simulink model "k6jca_181230_SHERA_ARDUINO_Comparison"  (R2018b)
settings: Solver=ode45  StartTime=0.0  StopTime=9000  MaxStep=1  RelTol=1e-3  EnableMultiTasking=on
InitFcn:
  | D=30
settings Model: Creator=Dick  LastModifiedBy=Jeff
settings DataIOCC: LimitDataPoints=on  SaveFormat=Array  SaveOutput=off  SignalLogging=off  DSMLogging=off  SaveTime=off
settings OptimizationCC: LifeSpan=inf
settings DebuggingCC: SFUnexpectedBacktrackingDiag=warning  SFNoUnconditionalDefaultTransitionDiag=warning  SFExecutionAtInitializationDiag=none
settings HardwareCC: ProdBitPerPointer=32  ProdBitPerSizeT=32  ProdBitPerPtrDiffT=32  ProdLargestAtomicFloat=None  ProdIntDivRoundTo=Undefined  ProdEndianess=Unspecified  ProdWordSize=32  ProdHWDeviceType=32-bit Generic
settings ModelReferenceCC: PropagateSignalLabelsOutOfModel=off
settings SFSimCC: SimUseLocalCustomCode=off
settings RTWCC: RTWUseLocalCustomCode=off
settings CodeAppCC: StateflowObjectComments=on
settings GRTTargetCC: TargetLangStandard=C89/C90 (ANSI)  GeneratePreprocessorConditionals=Disable all
settings ConfigComp: CovMetricSettings=dw  CovHtmlReporting=on  CovSaveCumulativeToWorkspaceVar=on  CovSaveSingleToWorkspaceVar=on  CovExternalEMLEnable=off

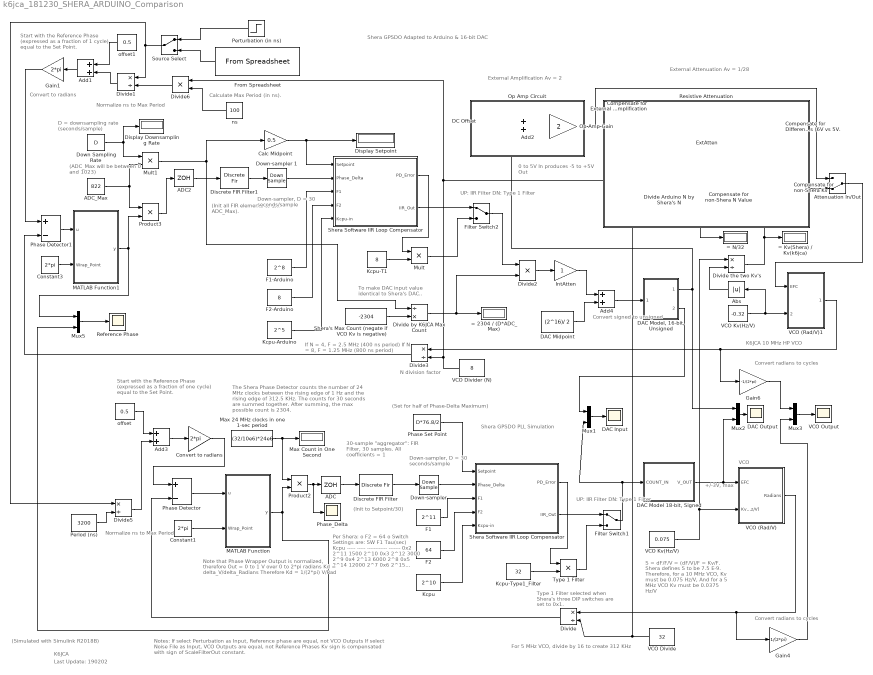
== system k6jca_181230_SHERA_ARDUINO_Comparison ==
  note: (Simulated with Simulink R2018B)
  note: Convert
      | signed
      | to unsigned
  note: To make DAC input value
      | identical to Shera's DAC..
  note: Notes:
      | If select Perturbation as Input, Reference phase are equal, not VCO Outputs
      | If select Noise File as Input, VCO Outputs are equal, not Reference Phases
      | Kv sign is compensated with sign of ScaleFilterOut constant.
  note: Normalize ns to
      | Max Period
  note: Calculate Max Period
      | (in ns).
  note: Down-sampler,
      | D = 30
      | seconds/sample
  note: Last Update: 190202
  note: (Set for half of Phase-Delta Maximum)
  note: 30-sample "aggregator":
      | FIR Filter,
      | 30 samples.
      | All coefficients = 1
  note: Start with the Reference Phase
      | (expressed as a fraction of one cycle)
      | equal to the Set Point.
  note: UP:  IIR Filter
      | DN:  Type 1 Filter
  note: Type 1 Filter selected
      | when Shera's three
      | DIP switches are set to 0x1.
  note: S = dF/F/V = (dF/V)/F = Kv/F.
      | Shera defines S to be 7.5 E-9.
      | Therefore, for a 10 MHz VCO,
      | Kv must be 0.075 Hz/V,
      | And for a 5 MHz VCO
      | Kv must be 0.0375 Hz/V
  note: The Shera Phase Detector counts the number of 24 MHz clocks between the rising edge of 1 Hz and the rising edge of 312.5 KHz.
      |
      | The counts for 30 seconds are summed together.  After summing,  the max possible count is 2304.
  note: Per Shera:
      |      o  F2 = 64
      |      o  Switch Settings are:
      |
      |    SW      F1     Tau(sec)    Kcpu
      |    -----     -----    ------------   -------
      |    0x2     2^11      1500       2^10
      |    0x3     2^12      3000       2^9
      |    0x4     2^13      6000       2^8
      |    0x5     2^14    12000       2^7
      |    0x6     2^15    24000       2^6
      |    0x7     2^16    48000       2^5
  note: For 5 MHz VCO, divide by 16 to create 312 KHz
  note: +/-3V,
      |  max
  note: K6JCA
  note: Shera GPSDO
      | PLL Simulation
  note: Convert radians to cycles
  note: Note that Phase Wrapper Output is normalized,
      | therefore Out =  0 to 1 V over 0 to 2*pi radians
      |
      | Kd = delta_V/delta_Radians
      | Therefore Kd = 1/(2*pi)  V/Rad
  note: VCO
  note: (Init to Setpoint/30)
  note: Convert to radians
  note: N division factor
  note: 0 to 5V In produces
      |  -5 to +5V Out
  note: External Attenuation
      | Av = 1/28
  note: D = downsampling rate
      |      (seconds/sample)
  note: If N = 4, F = 2.5 MHz   (400 ns period)
      | If N = 8, F = 1.25 MHz (800 ns period)
  note: (Init all FIR
      | elements to
      | 1/2 ADC_Max).
  note: (ADC_Max will be between 0 and 1023)
  note: Convert radians to cycles
  note: K6JCA 10 MHz HP VCO
  note: UP:  IIR Filter
      | DN:  Type 1 Filter
  note: Shera GPSDO Adapted
      | to Arduino & 16-bit DAC
  note: Start with the Reference Phase
      | (expressed as a fraction of 1 cycle)
      | equal to the Set Point.
  note: Normalize ns to
      | Max Period
  note: External Amplification
      | Av = 2
  note: Down-sampler,
      | D = 30
      | seconds/sample
  = 2304 / (D*ADC_Max) : Display
  = Kv(Shera) / Kv(k6jca) : Display
  = N/32 : Display
  ADC : ZeroOrderHold
  ADC2 : ZeroOrderHold
  ADC_Max : Constant  Value=822  SampleTime=Inf
  Abs : Abs
  Add{1..4} (4 alike) : Sum
  Attenuation In/Out : ManualSwitch  CurrentSetting=0
  Calc Midpoint : Gain  Gain=0.5
  "Compensate for non-Shera N Value " : Product  Inputs=**
  Compensate for non-Shera Kv : Product  Inputs=**
  Compensate for Different DAC ranges (6V vs 5V. : Gain  Gain=6/5
  Compensate for External Amplification : Gain  Gain=0.5
  Constant1 : Constant  Value=2*pi  SampleTime=Inf
  Constant3 : Constant  Value=2*pi
  "Convert to radians " : Gain  Gain=2*pi
  DAC Input : Scope
  DAC Midpoint : Constant  Value=(2^16)/ 2  SampleTime=Inf
  "DAC Model 18-bit, Signed" : Subsystem
  "DAC Model, 16-bit, Unsigned" : Subsystem
  DAC Output : Scope
  DC Offset : Constant  Value=-2.5  SampleTime=Inf
  Discrete FIR Filter : DiscreteFir  Coefficients=[1 1 1 1 1 1 1 1 1 1 1 1 1 1 1 1 1 1 1 1 1 1 1 1 1 1 1 1 1 1]  InitialStates=76.8/2
  Discrete FIR Filter1 : DiscreteFir  Coefficients=[1 1 1 1 1 1 1 1 1 1 1 1 1 1 1 1 1 1 1 1 1 1 1 1 1 1 1 1 1 1]  InitialStates=411
  "Display Downsampling Rate " : Display
  Display Setpoint : Display
  Divide{,1,3,5} (4 alike) : Product  Inputs=*/
  "Divide Arduino N by Shera's N " : Product  Inputs=*/
  Divide by K6JCA Max Count : Product  Inputs=/*
  Divide the two Kv's : Product  Inputs=*/
  Divide2 : Product  Inputs=**
  Divide6 : Product  Inputs=**
  "Down Sampling Rate " : Constant  Value=D  SampleTime=D
  "Down-sampler " : DownSample  N=D  RateOptions=Allow multirate processing
  Down-sampler 1 : DownSample  N=D  RateOptions=Allow multirate processing
  ExtAtten : Gain
  F1 : Constant  Value=2^11  SampleTime=Inf
  F1-Arduino : Constant  Value=2^8  SampleTime=Inf
  F2 : Constant  Value=64  SampleTime=Inf
  F2-Arduino : Constant  Value=8  SampleTime=Inf
  Filter Switch1 : ManualSwitch
  Filter Switch2 : ManualSwitch
  From Spreadsheet : FromSpreadsheet  FileName=Trimble_PD_181227.xlsx  SheetName=Sheet3
  Gain1 : Gain  Gain=2*pi
  Gain4 : Gain  Gain=1/(2*pi)
  Gain6 : Gain  Gain=-1/(2*pi)
  IntAtten : Gain
  Kcpu : Constant  Value=2^10  SampleTime=Inf
  Kcpu-Arduino : Constant  Value=2^5  SampleTime=Inf
  Kcpu-T1 : Constant  Value=8  SampleTime=Inf
  Kcpu-Type1_Filter : Constant  Value=32  SampleTime=Inf
  MATLAB Function : MATLAB Function  TreatAsAtomicUnit=on
  MATLAB Function1 : MATLAB Function  TreatAsAtomicUnit=on
  Max 24 MHz clocks in one 1-sec period : Constant  Value=(32/10e6)*24e6  SampleTime=Inf
  Max Count in One Second : Display
  Mult : Product  Inputs=**
  Mult1 : Product  Inputs=**
  Mux{1..3,5} (4 alike) : Mux  Inputs=2
  Op Amp Circuit : Subsystem
      mask Display: disp('')
  Op Amp Gain : Gain  Gain=2
  Period (ns) : Constant  Value=3200  SampleTime=Inf
  Perturbation (in ns) : Step  Time=100  After=400  SampleTime=1
  Phase Detector : Sum  Inputs=+-
  Phase Detector1 : Sum  Inputs=+-
  Phase Set Point : Constant  Value=D*76.8/2  SampleTime=Inf
  Phase_Delta : Scope
  Product2 : Product
  Product3 : Product
  Reference Phase : Scope
  Resistive Attenuation : Subsystem
      mask Display: disp('')
  Shera Software IIR Loop Compensator : Subsystem
  "Shera Software IIR Loop Compensator " : Subsystem
  Shera's Max Count (negate if VCO Kv is negative) : Constant  Value=-2304  SampleTime=Inf
  Source Select : ManualSwitch
  Type 1 Filter : Product  Inputs=**
  VCO (Rad/V) : Subsystem
  VCO (Rad/V)1 : Subsystem
  VCO Divide : Constant  Value=32  SampleTime=Inf
  VCO Divider (N) : Constant  Value=8  SampleTime=Inf
  VCO Kv(Hz/V) : Constant  Value=-0.32  SampleTime=Inf
  "VCO Kv(Hz/V) " : Constant  Value=0.075  SampleTime=Inf
  VCO Output : Scope
  ns : Constant  Value=100  SampleTime=Inf
  offset : Constant  Value=0.5  SampleTime=Inf
  offset1 : Constant  Value=0.5  VectorParams1D=off  SampleTime=Inf
  wires:
  Phase Detector/1 -> MATLAB Function/1(u)
  Constant1/1 -> MATLAB Function/2(Wrap_Point)
  Product2/1 -> Phase_Delta/1, ADC/1
  "Convert to radians "/1 -> Phase Detector/1
  "Shera Software IIR Loop Compensator "/1("PD_Error ") -> Type 1 Filter/1
  VCO (Rad/V)/1(Radians) -> Divide/1, Gain4/1
  F2/1 -> "Shera Software IIR Loop Compensator "/4(F2)
  F1/1 -> "Shera Software IIR Loop Compensator "/3(F1)
  Kcpu/1 -> "Shera Software IIR Loop Compensator "/5(Kcpu-in)
  "VCO Kv(Hz/V) "/1 -> VCO (Rad/V)/2(Kv_(Hz/V)), Divide the two Kv's/1
  "DAC Model 18-bit, Signed"/1(V_OUT) -> VCO (Rad/V)/1(EFC), Mux2/2
  Filter Switch1/1 -> Mux1/2, "DAC Model 18-bit, Signed"/1(COUNT_IN)
  Kcpu-Type1_Filter/1 -> Type 1 Filter/2
  Type 1 Filter/1 -> Filter Switch1/2
  "Shera Software IIR Loop Compensator "/2("IIR_Out ") -> Filter Switch1/1
  Phase Set Point/1 -> "Shera Software IIR Loop Compensator "/1(Setpoint)
  "Down-sampler "/1 -> "Shera Software IIR Loop Compensator "/2(Phase_Delta)
  Discrete FIR Filter/1 -> "Down-sampler "/1
  ADC/1 -> Discrete FIR Filter/1
  offset/1 -> Add3/1
  Divide/1 -> Phase Detector/2
  MATLAB Function/1(y) -> Mux5/2, Product2/2
  Max 24 MHz clocks in one 1-sec period/1 -> Max Count in One Second/1, Product2/1
  Add3/1 -> "Convert to radians "/1
  Divide5/1 -> Add3/2
  Period (ns)/1 -> Divide5/2
  VCO (Rad/V)1/1(Radians) -> Gain6/1, Divide3/1
  "Compensate for non-Shera N Value "/1 -> Compensate for non-Shera Kv/1
  Down-sampler 1/1 -> Shera Software IIR Loop Compensator/2(Phase_Delta)
  offset1/1 -> Add1/1
  Filter Switch2/1 -> Divide2/1
  "DAC Model, 16-bit, Unsigned"/1(V_OUT) -> Mux2/1, Add2/2
  Gain1/1 -> Phase Detector1/1
  ADC_Max/1 -> Mult1/2, Product3/1
  VCO Divide/1 -> "Divide Arduino N by Shera's N "/2, Divide/2
  Add2/1 -> Op Amp Gain/1
  Phase Detector1/1 -> MATLAB Function1/1(u)
  F1-Arduino/1 -> Shera Software IIR Loop Compensator/3(F1)
  Kcpu-Arduino/1 -> Shera Software IIR Loop Compensator/5(Kcpu-in)
  DC Offset/1 -> Add2/1
  Compensate for External Amplification/1 -> ExtAtten/1
  "Divide Arduino N by Shera's N "/1 -> "Compensate for non-Shera N Value "/2, = N/32/1
  Shera Software IIR Loop Compensator/2("IIR_Out ") -> Filter Switch2/1
  Product3/1 -> ADC2/1
  Shera Software IIR Loop Compensator/1("PD_Error ") -> Mult/1
  Kcpu-T1/1 -> Mult/2
  VCO Kv(Hz/V)/1 -> Abs/1, VCO (Rad/V)1/2(Kv_(Hz/V))
  ADC2/1 -> Discrete FIR Filter1/1
  Divide3/1 -> Phase Detector1/2
  Constant3/1 -> MATLAB Function1/2(Wrap_Point)
  Mult/1 -> Filter Switch2/2
  Compensate for Different DAC ranges (6V vs 5V./1 -> "Compensate for non-Shera N Value "/1
  "Down Sampling Rate "/1 -> "Display Downsampling Rate "/1, Mult1/1
  VCO Divider (N)/1 -> Divide3/2, "Divide Arduino N by Shera's N "/1, Divide6/1
  F2-Arduino/1 -> Shera Software IIR Loop Compensator/4(F2)
  ExtAtten/1 -> Compensate for Different DAC ranges (6V vs 5V./1
  Discrete FIR Filter1/1 -> Down-sampler 1/1
  Add1/1 -> Gain1/1
  Mux5/1 -> Reference Phase/1
  Mux2/1 -> DAC Output/1
  Gain6/1 -> Mux3/1
  Mux3/1 -> VCO Output/1
  Gain4/1 -> Mux3/2
  Divide1/1 -> Add1/2
  From Spreadsheet/1 -> Source Select/2
  Divide6/1 -> Divide1/2
  ns/1 -> Divide6/2
  Source Select/1 -> Divide1/1, Divide5/1
  Perturbation (in ns)/1 -> Source Select/1
  Divide the two Kv's/1 -> Compensate for non-Shera Kv/2, = Kv(Shera) / Kv(k6jca)/1
  Abs/1 -> Divide the two Kv's/2
  Divide2/1 -> IntAtten/1
  Mux1/1 -> DAC Input/1
  "DAC Model, 16-bit, Unsigned"/2(Quant_OUT1) -> Mux1/1
  MATLAB Function1/1(y) -> Mux5/1, Product3/2
  Op Amp Gain/1 -> Attenuation In/Out/1, Compensate for External Amplification/1
  Attenuation In/Out/1 -> VCO (Rad/V)1/1(EFC)
  Compensate for non-Shera Kv/1 -> Attenuation In/Out/2
  Add4/1 -> "DAC Model, 16-bit, Unsigned"/1(COUNT_IN)
  IntAtten/1 -> Add4/1
  DAC Midpoint/1 -> Add4/2
  Calc Midpoint/1 -> Shera Software IIR Loop Compensator/1(Setpoint), Display Setpoint/1
  Mult1/1 -> Calc Midpoint/1, Divide by K6JCA Max Count/1
  Shera's Max Count (negate if VCO Kv is negative)/1 -> Divide by K6JCA Max Count/2
  Divide by K6JCA Max Count/1 -> Divide2/2, = 2304 / (D*ADC_Max)/1

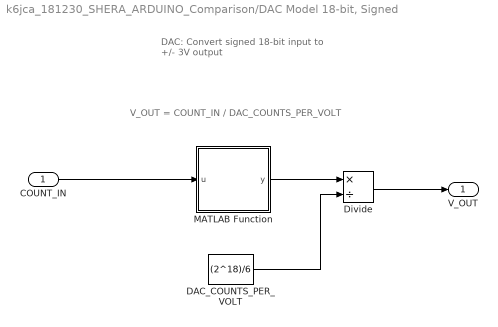
== system k6jca_181230_SHERA_ARDUINO_Comparison/DAC Model 18-bit, Signed ==
  note: V_OUT = COUNT_IN / DAC_COUNTS_PER_VOLT
  note: DAC:
      | Convert signed 18-bit input
      | to
      | +/- 3V output
  COUNT_IN : Inport
  "DAC_COUNTS_PER_VOLT " : Constant  Value=(2^18)/6  SampleTime=Inf
  Divide : Product  Inputs=*/
  MATLAB Function : MATLAB Function  TreatAsAtomicUnit=on
  V_OUT : Outport
  wires:
  "DAC_COUNTS_PER_VOLT "/1 -> Divide/2
  Divide/1 -> V_OUT/1
  MATLAB Function/1(y) -> Divide/1
  COUNT_IN/1 -> MATLAB Function/1(u)

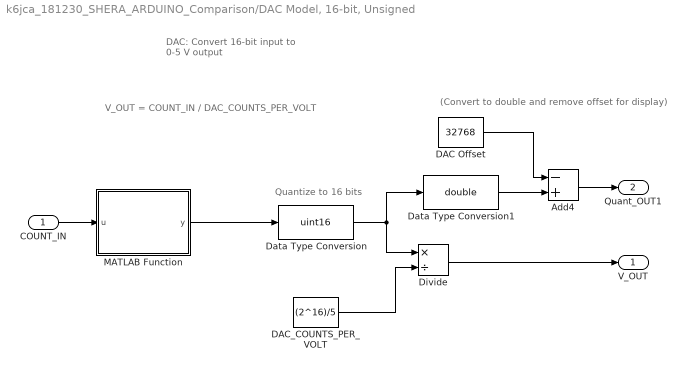
== system k6jca_181230_SHERA_ARDUINO_Comparison/DAC Model, 16-bit, Unsigned ==
  note: (Convert to double and remove offset for display)
  note: Quantize to 16 bits
  note: V_OUT = COUNT_IN / DAC_COUNTS_PER_VOLT
  note: DAC:
      | Convert 16-bit input
      | to
      | 0-5 V output
  COUNT_IN : Inport
  Add4 : Sum  Inputs=-+
  DAC Offset : Constant  Value=32768  SampleTime=Inf
  "DAC_COUNTS_PER_VOLT " : Constant  Value=(2^16)/5  SampleTime=Inf
  Data Type Conversion : DataTypeConversion  OutDataTypeStr=uint16
  Data Type Conversion1 : DataTypeConversion  OutDataTypeStr=double
  Divide : Product  Inputs=*/
  MATLAB Function : MATLAB Function  TreatAsAtomicUnit=on
  V_OUT : Outport
  Quant_OUT1 : Outport  Port=2
  wires:
  "DAC_COUNTS_PER_VOLT "/1 -> Divide/2
  Divide/1 -> V_OUT/1
  COUNT_IN/1 -> MATLAB Function/1(u)
  MATLAB Function/1(y) -> Data Type Conversion/1
  Data Type Conversion/1 -> Divide/1, Data Type Conversion1/1
  Add4/1 -> Quant_OUT1/1
  Data Type Conversion1/1 -> Add4/2
  DAC Offset/1 -> Add4/1

== system k6jca_181230_SHERA_ARDUINO_Comparison/Op Amp Circuit ==

== system k6jca_181230_SHERA_ARDUINO_Comparison/Resistive Attenuation ==

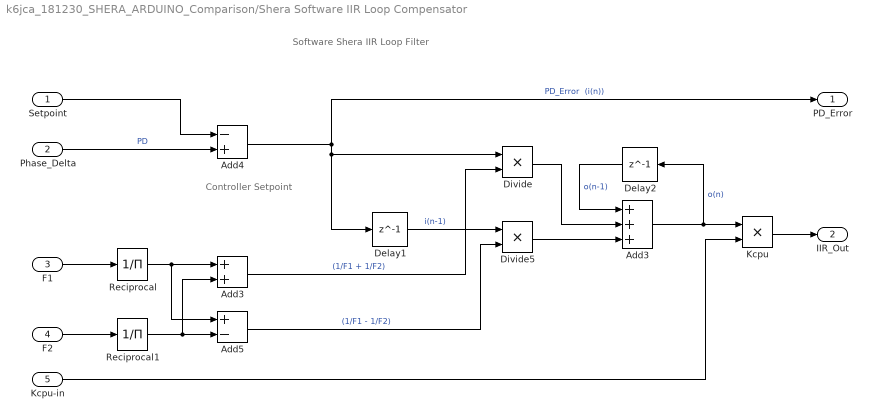
== system k6jca_181230_SHERA_ARDUINO_Comparison/Shera Software IIR Loop Compensator ==
  note: Software Shera IIR Loop Filter
  note: Controller
      | Setpoint
  Setpoint : Inport
  Phase_Delta : Inport  Port=2
  F1 : Inport  Port=3
  F2 : Inport  Port=4
  Kcpu-in : Inport  Port=5
  Add3 : Sum
  "Add3 " : Sum  Inputs=+++
  Add4 : Sum  Inputs=-+
  Add5 : Sum  Inputs=+-
  Delay1 : Delay  DelayLength=1
  Delay2 : Delay  DelayLength=1
  Divide : Product  Inputs=**
  Divide5 : Product  Inputs=**
  Kcpu : Product  Inputs=**
  Reciprocal : Product  Inputs=/
  Reciprocal1 : Product  Inputs=/
  "PD_Error " : Outport
  "IIR_Out " : Outport  Port=2
  wires:
  Setpoint/1 -> Add4/1
  Add4/1 -> Divide/1, Delay1/1, "PD_Error "/1  "PD_Error  (i(n))"
  "Add3 "/1 -> Delay2/1, Kcpu/1  "o(n)"
  F1/1 -> Reciprocal/1
  F2/1 -> Reciprocal1/1
  Reciprocal/1 -> Add5/1, Add3/1
  Reciprocal1/1 -> Add5/2, Add3/2
  Add3/1 -> Divide/2  "(1/F1 + 1/F2)"
  Delay1/1 -> Divide5/1  "i(n-1)"
  Add5/1 -> Divide5/2  "(1/F1 - 1/F2)"
  Delay2/1 -> "Add3 "/1  "o(n-1)"
  Divide/1 -> "Add3 "/2
  Divide5/1 -> "Add3 "/3
  Phase_Delta/1 -> Add4/2  "PD"
  Kcpu-in/1 -> Kcpu/2
  Kcpu/1 -> "IIR_Out "/1

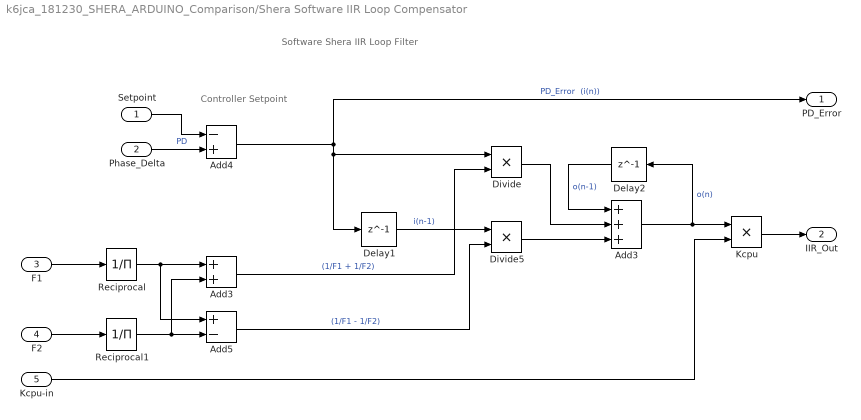
== system k6jca_181230_SHERA_ARDUINO_Comparison/Shera Software IIR Loop Compensator  ==
  note: Software Shera IIR Loop Filter
  note: Controller
      | Setpoint
  Setpoint : Inport
  Phase_Delta : Inport  Port=2
  F1 : Inport  Port=3
  F2 : Inport  Port=4
  Kcpu-in : Inport  Port=5
  Add3 : Sum
  "Add3 " : Sum  Inputs=+++
  Add4 : Sum  Inputs=-+
  Add5 : Sum  Inputs=+-
  Delay1 : Delay  DelayLength=1
  Delay2 : Delay  DelayLength=1
  Divide : Product  Inputs=**
  Divide5 : Product  Inputs=**
  Kcpu : Product  Inputs=**
  Reciprocal : Product  Inputs=/
  Reciprocal1 : Product  Inputs=/
  "PD_Error " : Outport
  "IIR_Out " : Outport  Port=2
  wires:
  Setpoint/1 -> Add4/1
  Add4/1 -> Divide/1, Delay1/1, "PD_Error "/1  "PD_Error  (i(n))"
  "Add3 "/1 -> Delay2/1, Kcpu/1  "o(n)"
  F1/1 -> Reciprocal/1
  F2/1 -> Reciprocal1/1
  Reciprocal/1 -> Add5/1, Add3/1
  Reciprocal1/1 -> Add5/2, Add3/2
  Add3/1 -> Divide/2  "(1/F1 + 1/F2)"
  Delay1/1 -> Divide5/1  "i(n-1)"
  Add5/1 -> Divide5/2  "(1/F1 - 1/F2)"
  Delay2/1 -> "Add3 "/1  "o(n-1)"
  Divide/1 -> "Add3 "/2
  Divide5/1 -> "Add3 "/3
  Phase_Delta/1 -> Add4/2  "PD"
  Kcpu-in/1 -> Kcpu/2
  Kcpu/1 -> "IIR_Out "/1

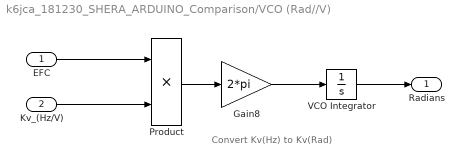
== system k6jca_181230_SHERA_ARDUINO_Comparison/VCO (Rad//V) ==
  note: Convert Kv(Hz)
      | to Kv(Rad)
  EFC : Inport
  Kv_(Hz/V) : Inport  Port=2
  Gain8 : Gain  Gain=2*pi
  Product : Product
  VCO Integrator : Integrator
  Radians : Outport
  wires:
  Gain8/1 -> VCO Integrator/1
  EFC/1 -> Product/1
  Product/1 -> Gain8/1
  VCO Integrator/1 -> Radians/1
  Kv_(Hz/V)/1 -> Product/2

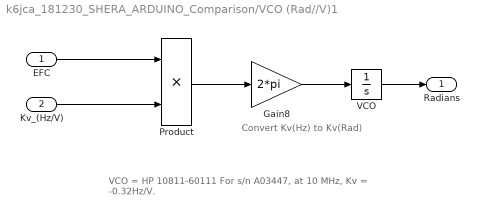
== system k6jca_181230_SHERA_ARDUINO_Comparison/VCO (Rad//V)1 ==
  note: VCO = HP 10811-60111
      |
      | For s/n A03447, at 10 MHz, Kv = -0.32Hz/V.
  note: Convert Kv(Hz)
      | to Kv(Rad)
  EFC : Inport
  Kv_(Hz/V) : Inport  Port=2
  Gain8 : Gain  Gain=2*pi
  Product : Product
  VCO : Integrator
  Radians : Outport
  wires:
  Gain8/1 -> VCO/1
  EFC/1 -> Product/1
  Product/1 -> Gain8/1
  VCO/1 -> Radians/1
  Kv_(Hz/V)/1 -> Product/2

== matlab function k6jca_181230_SHERA_ARDUINO_Comparison/MATLAB Function ==
  data: u input; y output; Wrap_Point input
function y = phase_wrapper(u,Wrap_Point)
%#codegen
y=0;
if u > 0
   y = mod(u,Wrap_Point);
elseif u < 0
   y = Wrap_Point-(mod(-u,Wrap_Point));  
end
y = y/Wrap_Point;  % normalize y to 1.

== matlab function k6jca_181230_SHERA_ARDUINO_Comparison/DAC Model 18-bit, Signed/MATLAB Function ==
  data: u input; y output
function y = dac_limiter(u)
%#codegen
% This limits the DAC input to +131071
% and to -131072 (18 bit range).

y = u;
if u > 131071
   y = 131071;
elseif u < -131072
   y = -131072;  
end

== matlab function k6jca_181230_SHERA_ARDUINO_Comparison/MATLAB Function1 ==
  data: u input; y output; Wrap_Point input
function y = phase_wrapper(u,Wrap_Point)
%#codegen
y=0;
if u > 0
   y = mod(u,Wrap_Point);
elseif u < 0
   y = Wrap_Point-(mod(-u,Wrap_Point));  
end
y = y/Wrap_Point;  % normalize y to 1.

== matlab function k6jca_181230_SHERA_ARDUINO_Comparison/DAC Model, 16-bit, Unsigned/MATLAB Function ==
  data: y output; u input
function y = b16_dac_limiter(u)
%#codegen
% This limits the DAC input to 65535 and 0
%
y = u;
if u > 65535
   y = 65535;
elseif u < 0
   y = 0;  
end
